simulink model "Simulink_Practica1_v2019"  (R2020b)
settings: Solver=FixedStepDiscrete  StartTime=0.0  StopTime=inf  FixedStep=0.01  RelTol=1e-3  EnableMultiTasking=on
libraries: instrumentlib x2, sldrtlib x1, aerolibanimutils x1
settings Model: Creator=Usuario  LastModifiedBy=Agustin
settings DataIOCC: LimitDataPoints=on  SaveFormat=Array  ReturnWorkspaceOutputs=off
settings OptimizationCC: LifeSpan=inf
settings DebuggingCC: SolverPrmCheckMsg=warning  SFUnexpectedBacktrackingDiag=warning  SFNoUnconditionalDefaultTransitionDiag=warning  ArithmeticOperatorsInVariantConditions=warning
settings HardwareCC: ProdBitPerPointer=32  ProdBitPerSizeT=32  ProdBitPerPtrDiffT=32  ProdLargestAtomicFloat=None  ProdIntDivRoundTo=Undefined  ProdEndianess=Unspecified  ProdWordSize=32  ProdHWDeviceType=32-bit Generic
settings ModelReferenceCC: PropagateSignalLabelsOutOfModel=off
settings SFSimCC: SimUseLocalCustomCode=off  CustomCodeUndefinedFunction=UseInterfaceOnly
settings RTWCC: RTWUseLocalCustomCode=off
settings CodeAppCC: StateflowObjectComments=on
settings GRTTargetCC: TargetLangStandard=C89/C90 (ANSI)
settings ConfigComp: CovMetricSettings=dw  CovSaveCumulativeToWorkspaceVar=on  CovSaveSingleToWorkspaceVar=on  CovExternalEMLEnable=off  CovSFcnEnable=off

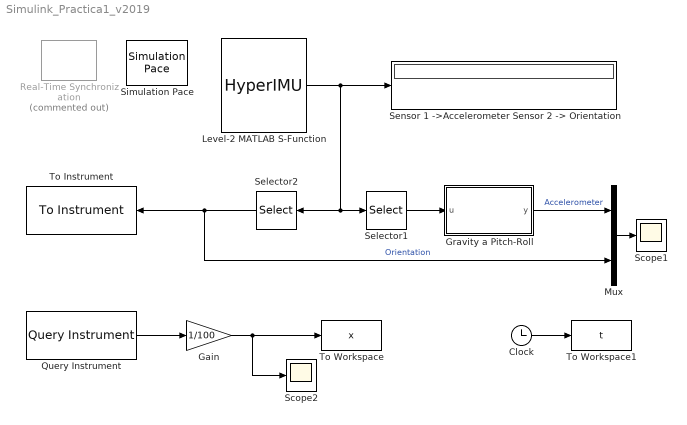
== system Simulink_Practica1_v2019 ==
  Clock : Clock
  Gain : Gain  Gain=1/100
  Gravity a Pitch-Roll : MATLAB Function  TreatAsAtomicUnit=on
  Level-2 MATLAB S-Function : M-S-Function  FunctionName=HyperIMU  Parameters=NoS,PN,ST  mask(HyperIMU){NoS=2, PN=2055, ST=0.03}
      mask prompts: NoS "Nº of Sensors"; PN "Port Number"; ST "Sample Time"
      mask help: Bloque que recibe datos de la app HyperIMU (protocolo UDP). Los parámetros a setear indican la cantidad de sensores, el número de puerto y el tiempo de muestreo, todos los parámetros deben coincidir con la configuración de la app en el celular.
      mask Display: image('HyperImu.png')
  Mux : Mux  Inputs=2
  Query Instrument : instrumentlib/Query Instrument  sampleTime=0.01  isWorkspaceObject=off  timeout=10  inputBufferSize=512  protocol=Serial  serialPort=COM4  baudRate=115200  gpibVendor=Keysight Technologies  boardIndex=0  primaryAddress=1  secondaryAddress=0  visaVendor=Keysight  visaSerialPort=0  chassisIndex=0  logicalAddress=0  tcpRemoteHost='127.0.0.1'  tcpRemotePort=4500  udpRemoteHost='127.0.0.1'  udpRemotePort=9090  visaTCPBoardIndex=0  visaTCPRemoteHost='127.0.0.1'  usbBoardIndex=0  usbManufID=0  usbModelCode=0  usbSerialNumber=0  initAction=None  initCommand='DATA:SOURCE CH1'  initFunction=get  queryCommand=''  responseFormat=ASCII  asciiFormatting='%d,%d,%d,%d'  precision=8-bit integer  byteOrder=Little endian  valuesToRead=1  removeBytes=off  afterOutputAction=Repeat query for new data  enableFrames=on  frameSize=4
      settings: SourceProductBaseCode=IC
  Real-Time Synchronization : sldrtlib/Real-Time Synchronization  Commented=on  SampleTime=0.01  MaxMissedTicks=inf  ShowMissedTicks=off  YieldWhenWaiting=off
  Scope1 : Scope
  Scope2 : Scope
  Selector1 : Selector  NumberOfDimensions=2  IndexOptions=Index vector (dialog),Starting index (dialog)  Indices=1,1  OutputSizes=1,3
  Selector2 : Selector  NumberOfDimensions=2  IndexOptions=Index vector (dialog),Starting index (dialog)  Indices=2,3  OutputSizes=1,1
  "Sensor 1 ->Accelerometer Sensor 2 -> Orientation" : Display
  Simulation Pace : aerolibanimutils/Simulation Pace  SimulationPace=1  SleepMode=MATLAB Thread  OutputPaceError=off  SampleTime=-1
  To Instrument : instrumentlib/To Instrument  sampleTime=-1  isWorkspaceObject=off  timeout=10  inputBufferSize=512  protocol=Serial  serialPort=COM4  baudRate=115200  gpibVendor=ICS Electronics  boardIndex=0  primaryAddress=1  secondaryAddress=0  visaVendor=Keysight  visaSerialPort=0  chassisIndex=0  logicalAddress=0  tcpRemoteHost='127.0.0.1'  tcpRemotePort=4500  udpRemoteHost='127.0.0.1'  udpRemotePort=9090  visaTCPBoardIndex=0  visaTCPRemoteHost='127.0.0.1'  usbBoardIndex=0  usbManufID=0  usbModelCode=0  usbSerialNumber=0  initAction=None  initCommand='DATA:SOURCE CH1'  initFunction=get  command=''  sendFormat=ASCII  asciiFormatting='%f\n'  precision=16-bit integer  byteOrder=Little endian
      settings: SourceProductBaseCode=IC
  To Workspace : ToWorkspace  VariableName=x  SampleTime=-1
  To Workspace1 : ToWorkspace  VariableName=t  SampleTime=-1
  wires:
  Clock/1 -> To Workspace1/1
  Query Instrument/1 -> Gain/1
  Gain/1 -> Scope2/1, To Workspace/1
  Selector2/1 -> Mux/2, To Instrument/1  "Orientation"
  Level-2 MATLAB S-Function/1 -> Selector2/1, Selector1/1, "Sensor 1 ->Accelerometer Sensor 2 -> Orientation"/1
  Selector1/1 -> Gravity a Pitch-Roll/1(u)
  Gravity a Pitch-Roll/1(y) -> Mux/1  "Accelerometer"
  Mux/1 -> Scope1/1

== matlab function Simulink_Practica1_v2019/Gravity a Pitch-Roll ==
  data: u input; y output
function y = fcn(u)
Gx=u(1);
Gy=u(2);
Gz=u(3);
roll = rad2deg(atan2(Gy,Gz));
pitch = rad2deg(atan2(-Gx,sqrt(Gy*Gy+Gz*Gz)));

y = -pitch;
